simulink library "Lib_EMTAT"  (R2021b)
settings: Solver=VariableStepAuto  StartTime=0.0  StopTime=10.0  RelTol=1e-3
undefined symbols (not defined in the file or in its folder): A_M, B_M, Cj, component_degradation_input, Cs, E0_M, f_sw, K_M, MWS, Q_M, Q_rr, r_c, r_D, R_M, Rj, Ru, SNR_DX_M, SNR_IC_M, SNR_Mn_M, SNR_Mx_M, SOC_Init_M, u_ce0, u_D0
libraries: $bdroot x82, simulink x23, Lib_Dyn_StateSpace_EMTAT x3, PB_Library_Master_Working x1
(part 3 of 7)

== system Lib_EMTAT/Components/Power Flow ==
  note: Add efficiency tables to converters, inverter, and rectifier.
  note: [gcb '/Deg']
  AC-AC Transformer : Subsystem  mask(AC/AC Transformer){X_C_VoltageAC1Vec_M=MWS.I1.Vdc, Y_C_CurrentAC2Vec_M=MWS.I1.Irms, T_C_PowLossArray_M=MWS.I1.Ploss', K=0.0503, FM=0, Plosslim=0}
      mask prompts: X_C_VoltageAC1Vec_M "X_C_VoltageAC1Vec_M - Primary AC Line to Neutral RMS Voltage Vector (X-axis)(nx1)"; Y_C_CurrentAC2Vec_M "Y_C_CurrentAC2Vec_M - Secondary RMS Line Current Vector (Y-axis)(mx1)"; T_C_PowLossArray_M "T_C_PowLossArray_M - Power Loss Table Values (Ploss = f(Irmsout, Vin)(nxm)"; K "Transformer Ratio"; FM "Mode:"; Plosslim "Plosslim - Power Loss Limit, W"
      mask help: This block models an AC/AC transofrmer. The power through the transformer is modified by a user-input power loss table. The primary side is designated as 1. The secondary side is designated as 2.
      settings: AttributesFormatString=AC/AC Transformer
      mask Help:
      | Inputs:
      | 	V_LN_rms_1: Primary line to neutral root-mean-squared alternating current voltage, V_LN_rms (1x1)
      | 	I_L_rms_2: Secondary line root-mean-squared alternating current, A_L_rms (1x1)
      | 	Fail?: Failure toggle (0 = Not failed, 1 = Failed)
      | 	Deg: Decimal percantage of maximum power degredation (0 = New component, 1 = End of life component)
      | Mask Variables:
      | 	X_C_VoltageAC1Vec_M: Primary alternating current line to neutral root-mean-squared voltage vector for power loss map, V_LN_rms (nx1)
      | 	Y_C_CurrentAC2Vec_M: Secondary line root-mean-squared alternating current vector for power loss map, A_LN_rms (nx1)
      | 	T_C_PlossArray_M: Power loss map, W (nxm)
      | 	Failure Modes
      | 		1 - Open circuit.
      | 		2 - Degredation.
      | 	Plosslim: Maximum additional power loss, W (1x1)
      | Outputs:
      | 	V_LN_rms_2: Secondary line to neutral root-mean-squared alternating current voltage, V_LN_rms (1x1)
      | 	Outputs: Low level signals (Bus)
      | 		P_AC_2: Secondary side power, W (1x1)
      | 		P_AC_1: Primary Side power, W (1x1)
      | 		Eff: Efficiency, decimal percentage (1x1)
      | 		V_LN_rms_2: Secondary line to neutral root-mean-squared alternating current voltage, V_LN_rms (1x1)
      | 		V_LN_rms_1: Primary line to neutral root-mean-squared alternating current voltage, V_LN_rms (1x1)
      | 		I_L_rms_2: Secondary line root-mean-squared alternating current, A_L_rms (1x1)
      | 		I_L_rms_1: Primary line root-mean-squared alternating current, I_L_rms (1x1)
      | 		Ploss: Power loss, W (1x1)
      | 	Ploss: Power loss, W (1x1)
      | 	I_L_rms_1: Primary line root-mean-squared alternating current, I_L_rms (1x1)
      mask DialogControl Control3 Prompt: Plot Power Loss Map
      mask DialogControl Control3 Callback:
      | % Plot efficiency map.
      | vals = get_param(gcb,'MaskValues');
      | X = str2num(cell2mat(vals(1)));
      | Y = str2num(cell2mat(vals(2)));
      | Z = str2num(cell2mat(vals(3)));
      | [X,Y] = meshgrid(X,Y);
      | figure('name',[get_param(gcb,'name') ' Power Loss Map'],'numbertitle','off')
      | contour(X,Y,Z,15);
      | xlabel('Voltage In, VDC')
      | ylabel('Line Current Out, A_{rms}')
      | title([get_param(gcb,'name') ' Power Loss Map'])
      | c = colorbar;
      | c.Label.String = 'Power Loss, W';
      mask DialogControl Container3 Prompt: Failure Modes
      mask DialogControl Control2 Prompt: 1 - Open Circuit, 2 - Degradation
  AC-DC Rectifier : Subsystem  mask(Inverter/Rectifier (Source)){X_C_VoltageInVec_M=[0 1000], Y_C_RMSCurrentOutVec_M=[0 1000], T_C_PowLossArray_M=0*ones(2), FM=0, Plosslim=0}
      mask prompts: X_C_VoltageInVec_M "X_C_VoltageInVec_M - DC Voltage Vector (X-axis)(nx1)"; Y_C_RMSCurrentOutVec_M "Y_C_RMSCurrentOutVec_M - RMS Line Current Vector (Y-axis)(mx1)"; T_C_PowLossArray_M "T_C_PowLossArray_M - Power Loss Table Values (Ploss = f(Irmsout, Vin)(nxm)"; FM "Mode:"; Plosslim "Plosslim - Power Loss Limit, W"
      mask help: This block models an inverter/rectifier for use as a power source. The power through the inverter/rectifier is modified by a user-input power loss table.
      settings: AttributesFormatString=AC-DC Rectifier
      mask Help:
      | Inputs:
      | 	V_LN_rms: Line to neutral alternating current voltage, Vrms (1x1)
      | 	I_DC: Direct current, ADC (1x1)
      | 	Fail?: Failure toggle (0 = Not failed, 1 = Failed)
      | 	Deg: Decimal percantage of maximum power degredation (0 = New component, 1 = End of life component)
      | 	I_L_rms(t-1): Line alternating current from one time step delay block, Arms (1x1)
      | Mask Variables:
      | 	X_C_VoltageInVec_M: Direct current voltage vector for efficiency map, VDC (nx1)
      | 	Y_C_RMSCurrentOutVec_M: Line alternating current vector for efficiency map, Irms (mx1)
      | 	T_C_PowLossArray_M: Efficiency matrix, decimal % (nxm)
      | 	K_e: Peak line to line back electromotive force voltage, Vpeak (1x1)
      | 	Failure Modes
      | 		1 - Open circuit.
      | 		2 - Degredation.
      | 	Plosslim: Maximum additional power loss, W (1x1)
      | Outputs:
      | 	V_DC: Direct current voltage, VDC (1x1)
      | 	Outputs: Low level signals (Bus)
      | 		P_AC: Instantaneous alternating current power, W (1x1)
      | 		P_DC: Direct current power, W (1x1)
      | 		Eff: Efficiency, decimal % (1x1)
      | 		V_LN_rms: Line to neutral alternating current voltage, Vrms (1x1)
      | 		V_DC: Direct current voltage, VDC (1x1)
      | 		Vdot_DC: Derivative of direct current voltage, VDC/s (1x1)
      | 		I_L_rms: Line alternating current, Irms (1x1)
      | 		I_DC: Direct current, ADC (1x1)
      | 		Idot_DC: Derivative of direct current, ADC/s (1x1)
      | 		Ploss: Power loss, W (1x1)
      | 	Ploss: Power loss, W (1x1)
      | 	I_L_rms: Line alternating current, Arms (1x1)
      | 	I_L_rms(1): Line alternating current to one time step delay block, Arms (1x1)
      mask DialogControl Control2 Prompt: Plot Power Loss Map
      mask DialogControl Control2 Callback:
      | % Plot efficiency map.
      | vals = get_param(gcb,'MaskValues');
      | X = str2num(cell2mat(vals(1)));
      | Y = str2num(cell2mat(vals(2)));
      | Z = str2num(cell2mat(vals(3)));
      | [X,Y] = meshgrid(X,Y);
      | figure('name',[get_param(gcb,'name') ' Power Loss Map'],'numbertitle','off')
      | contour(X,Y,Z,15);
      | xlabel('Voltage In, VDC')
      | ylabel('Line Current Out, A_{rms}')
      | title([get_param(gcb,'name') ' Power Loss Map'])
      | c = colorbar;
      | c.Label.String = 'Power Loss, W';
      mask DialogControl Container3 Prompt: Failure Modes
      mask DialogControl Control3 Prompt: 1 - Open Circuit, 2 - Degradation
  Cable : Subsystem  mask(Cable){R=0.2}
      mask prompts: R "R_c - Resistance, Ohm"
      mask help: This block models a cable with resistive effects.
      settings: AttributesFormatString=Cable
      mask Help:
      | Inputs:
      | 	Vin: Input voltage, VDC (1x1)
      | 	Iout: Output current, ADC (1x1)
      | 	Fail?: Failure toggle (0 = Not failed, 1 = Failed)
      | 	Iout(t-1): Output curernt from one time step delay block, ADC (1x1)
      | Mask Variables:
      | 	R: Resistance, Ohm (1x1)
      | 	Failure Modes:
      | 		Open circuit failure.
      | Outputs:
      | 	Vout: Output voltage, VDC (1x1)
      | 	Outputs: Low level signals (Bus)
      | 		Pout: Electrical power out, W (1x1)
      | 		Pin: Electrical power in, W (1x1)
      | 		Iin: Input current, ADC (1x1)
      | 		Iout: Output current, ADC (1x1)
      | 		Vin: Input voltage, VDC (1x1)
      | 		Vout: Output voltage, VDC (1x1)
      | 		R: Resistance, Ohm (1x1)
      | 		Ploss: Power loss due to resistive effects, W (1x1)
      | 	Ploss: Power loss due to resistive effects, W (1x1)
      | 	Iin: Input current, ADC (1x1)
      | 	Iout(t): Output current to one time step delay block, ADC (1x1)
      mask DialogControl Container3 Prompt: Failure Modes
      mask DialogControl Control2 Prompt: Mode: Open Circuit
  Current Distribution : Subsystem  mask(Current Distribution){}
      settings: AttributesFormatString=Current Distribution
  Current Junction : Subsystem  mask(Current Junction){Nb=3}
      mask prompts: Nb "Nb - # of branches"
      mask help: This block adds a vector of input currents (I).
      settings: AttributesFormatString=Current Junction
      mask Help:
      | Inputs:
      | 	I: Currents to be summed, ADC (nx1)
      | Outputs:
      | 	Isum: Net current, ADC (1x1)
      mask DialogControl Control2 Prompt: Note: There is no limit to the number of multiplexed currents.
      mask DialogControl Container2 Prompt: Parameters
  DC-AC Inverter : Subsystem  mask(Inverter/Rectifier (Sink)){X_C_VoltageInVec_M=[0 1000], Y_C_RMSCurrentOutVec_M=[0 1000], T_C_PowLossArray_M=zeros(2), K_e=0.0503, FM=0, Plosslim=0}
      mask prompts: X_C_VoltageInVec_M "X_C_VoltageInVec_M - DC Voltage Vector (X-axis)(nx1)"; Y_C_RMSCurrentOutVec_M "Y_C_RMSCurrentOutVec_M - RMS Line Current Vector (Y-axis)(mx1)"; T_C_PowLossArray_M "T_C_PowLossArray_M - Power Loss Table Values (Ploss = f(Irmsout, Vin)(nxm)"; K_e "K_e - Back EMF Constant, V_LL_peak/RPM"; FM "Mode:"; Plosslim "Plosslim - Power Loss Limit, W"
      mask help: This block models an inverter/rectifier for use as a power sink. The power through the inverter/rectifier is modified by a user-input efficiency table.
      settings: AttributesFormatString=DC-AC Inverter
      mask Help:
      | Inputs:
      | 	V_DC: Direct current voltage, VDC (1x1)
      | 	N: Shaft speed, RPM (1x1)
      | 	I_L_rms: Line alternating current, Arms (1x1)
      | 	Fail?: Failure toggle (0 = Not failed, 1 = Failed)
      | 	Deg: Decimal percantage of maximum power degredation (0 = New component, 1 = End of life component)
      | Mask Variables:
      | 	X_C_VoltageInVec_M: Direct current voltage vector for efficiency map, VDC (nx1)
      | 	Y_C_RMSCurrentOutVec_M: Line alternating current vector for efficiency map, Irms (mx1)
      | 	T_C_PowLossArray_M: Efficiency matrix, decimal % (nxm)
      | 	K_e: Peak line to line back electromotive force voltage, Vpeak (1x1)
      | 	Failure Modes
      | 		1 - Open circuit.
      | 		2 - Degredation.
      | 	Plosslim: Maximum additional power loss, W (1x1)
      | Outputs:
      | 	V_LN_rms: Line to neutral alternating current voltage, Vrms (1x1)
      | 	Outputs: Low level signals (Bus)
      | 		P_AC: Instantaneous alternating current power, W (1x1)
      | 		P_DC: Direct current power, W (1x1)
      | 		Eff: Efficiency, decimal % (1x1)
      | 		V_LN_rms: Line to neutral alternating current voltage, Vrms (1x1)
      | 		V_DC: Direct current voltage, VDC (1x1)
      | 		Vdot_DC: Derivative of direct current voltage, VDC/s (1x1)
      | 		I_L_rms: Line alternating current, Irms (1x1)
      | 		I_DC: Direct current, ADC (1x1)
      | 		Idot_DC: Derivative of direct current, ADC/s (1x1)
      | 		Ploss: Power loss, W (1x1)
      | 	Ploss: Power loss, W (1x1)
      | 	I_DC: Direct current, ADC (1x1)
      mask DialogControl Control3 Prompt: Plot Power Loss Map
      mask DialogControl Control3 Callback:
      | % Plot efficiency map.
      | vals = get_param(gcb,'MaskValues');
      | X = str2num(cell2mat(vals(1)));
      | Y = str2num(cell2mat(vals(2)));
      | Z = str2num(cell2mat(vals(3)));
      | [X,Y] = meshgrid(X,Y);
      | figure('name',[get_param(gcb,'name') ' Power Loss Map'],'numbertitle','off')
      | contour(X,Y,Z,15);
      | xlabel('Voltage In, VDC')
      | ylabel('Line Current Out, A_{rms}')
      | title([get_param(gcb,'name') ' Power Loss Map'])
      | c = colorbar;
      | c.Label.String = 'Power Loss, W';
      mask DialogControl Container3 Prompt: Failure Modes
      mask DialogControl Control2 Prompt: 1 - Open Circuit, 2 - Degradation
  DC-DC Converter (Set Output Voltage) : Subsystem  mask(DC-DC Converter (Set Output Voltage)){X_Vin_VoltageVec_M=[0 100 1000 5000], Y_Iout_CurrentVec_M=[0 10 100 150], T_C_PlossArray_M=0.98*ones(4,4), FM=0, Plosslim=0}
      mask prompts: X_Vin_VoltageVec_M "X_Vin_VoltageVec_M - Efficiency Table Voltage In Vector (X-axis)(nx1)"; Y_Iout_CurrentVec_M "Y_Iout_CurrentVec_M - Efficiency Table Current Out Vector (Y-axis)(mx1)"; T_C_PlossArray_M "T_C_PlossArray_M - Power Loss Table Values (Eff = f(i, V)(nxm)"; FM "Mode:"; Plosslim "Plosslim - Power Loss Limit, W"
      mask help: This block models the power flow through a DC-DC converter using a user specified power loss table. The output voltage (Vout) can also be set using variable Vset.
      settings: AttributesFormatString=|
      | DC-DC Converter
      | (Set Output Voltage)
      mask Help:
      | Inputs:
      | 	Vset: Voltage setpoint, VDC (1x1)
      | 	Vin: Input voltage, VDC (1x1)
      | 	Iout: Output current, ADC (1x1)
      | 	Fail?: Failure toggle (0 = Not failed, 1 = Failed)
      | 	Deg: Decimal percantage of maximum power degredation (0 = New component, 1 = End of life component)
      | Mask Variables:
      | 	X_Vin_VoltageVec_M: Input voltage vector for power loss map, VDC (nx1)
      | 	Y_Iout_CurrentVec_M: Output current vector for power loss map, ADC (mx1)
      | 	T_C_PlossArray_M: Power loss map, W (nxm)
      | 	Failure Modes
      | 		1 - Open circuit.
      | 		2 - Degredation.
      | 	Plosslim: Maximum additional power loss, W (1x1)
      | Outputs:
      | 	Vout: Output voltage, VDC (1x1)
      | 	Outputs: Low level signals (Bus)
      | 		Pin: Input power, W (1x1)
      | 		Pout: Output power, W (1x1)
      | 		Eff: Efficiency, decimal % (1x1)
      | 		Vout: Output voltage, VDC (1x1)
      | 		Vdotout: Derivative of output voltage, VDC/s (1x1)
      | 		Vin: Input voltage, VDC (1x1)
      | 		Vdotin: Derivative of input voltage, VDC/s (1x1)
      | 		Iin: Input current, ADC (1x1)
      | 		Idotin: Derivative of input current, ADC/s (1x1)
      | 		Iout: Output current, ADC (1x1)
      | 		Idotout: Derivative of output current, ADC/s (1x1)
      | 		Ploss: Power loss, W (1x1)
      | 		Vset: Voltage setpoint, VDC (1x1)
      | 	Ploss: Power loss, W (1x1)
      | 	Iin: Input current, ADC (1x1)
      mask DialogControl Control3 Prompt: Plot Power Loss Map
      mask DialogControl Control3 Callback:
      | % Plot power loss map.
      | vals = get_param(gcb,'MaskValues');
      | X = str2num(cell2mat(vals(1)));
      | Y = str2num(cell2mat(vals(2)));
      | Z = str2num(cell2mat(vals(3)));
      | [X,Y] = meshgrid(X,Y);
      | figure('name',[get_param(gcb,'name') ' Power Loss Map'],'numbertitle','off')
      | contour(X,Y,Z,15);
      | xlabel('Voltage In, VDC')
      | ylabel('Current Out, ADC')
      | title([get_param(gcb,'name') ' Power Loss Map'])
      | c = colorbar;
      | c.Label.String = 'Power loss, W';
      mask DialogControl Container3 Prompt: Failure Modes
      mask DialogControl Control2 Prompt: 1 - Open Circuit, 2 - Degradation
  DC-DC Converter (Regulate Output Voltage) : Subsystem  mask(DC-DC Converter (Regulate Output Voltage)){X_Vin_VoltageVec_M=[0 100 1000 5000], Y_Iout_CurrentVec_M=[0 10 100 150], T_C_PlossArray_M=0.98*ones(4,4), FM=0, Plosslim=0}
      mask prompts: X_Vin_VoltageVec_M "X_Vin_VoltageVec_M - Efficiency Table Voltage In Vector (X-axis)(nx1)"; Y_Iout_CurrentVec_M "Y_Iout_CurrentVec_M - Efficiency Table Current Out Vector (Y-axis)(mx1)"; T_C_PlossArray_M "T_C_PlossArray_M - Power Loss Table Values (Eff = f(i, V)(nxm)"; FM "Mode:"; Plosslim "Plosslim - Power Loss Limit, W"
      mask help: This block models the power flow through a DC-DC converter using a user specified efficiency table. The output voltage (Vout) can also be set using variable Vset.
      settings: AttributesFormatString=|
      | DC-DC Converter
      | (Regulate Output Voltage)
      mask Help:
      | Inputs:
      | 	Vout: Output voltage, VDC (1x1)
      | 	Vin: Input voltage, VDC (1x1)
      | 	Ioutdmd: Output current demand, ADC (1x1)
      | 	Fail?: Failure toggle (0 = Not failed, 1 = Failed)
      | 	Deg: Decimal percantage of maximum power degredation (0 = New component, 1 = End of life component)
      | Mask Variables:
      | 	X_Vin_VoltageVec_M: Input voltage vector for power loss map, VDC (nx1)
      | 	Y_Iout_CurrentVec_M: Output current vector for power loss map, ADC (mx1)
      | 	T_C_PlossArray_M: Power loss map, W (nxm)
      | 	Failure Modes
      | 		1 - Open circuit.
      | 		2 - Degredation.
      | 	Plosslim: Maximum additional power loss, W (1x1)
      | Outputs:
      | 	Outputs: Low level signals (Bus)
      | 		Pin: Input power, W (1x1)
      | 		Pout: Output power, W (1x1)
      | 		Eff: Efficiency, decimal % (1x1)
      | 		Vout: Output voltage, VDC (1x1)
      | 		Vdotout: Derivative of output voltage, VDC/s (1x1)
      | 		Vin: Input voltage, VDC (1x1)
      | 		Vdotin: Derivative of input voltage, VDC/s (1x1)
      | 		Iin: Input current, ADC (1x1)
      | 		Idotin: Derivative of input current, ADC/s (1x1)
      | 		Iout: Output current, ADC (1x1)
      | 		Idotout: Derivative of output current, ADC/s (1x1)
      | 		Ploss: Power loss, W (1x1)
      | 	Ploss: Power loss, W (1x1)
      | 	Iin: Input current, ADC (1x1)
      | 	Iout: Output current, ADC (1x1)
      mask DialogControl Control3 Prompt: Plot Power Loss Map
      mask DialogControl Control3 Callback:
      | % Plot power loss map.
      | vals = get_param(gcb,'MaskValues');
      | X = str2num(cell2mat(vals(1)));
      | Y = str2num(cell2mat(vals(2)));
      | Z = str2num(cell2mat(vals(3)));
      | [X,Y] = meshgrid(X,Y);
      | figure('name',[get_param(gcb,'name') ' Power Loss Map'],'numbertitle','off')
      | contour(X,Y,Z,15);
      | xlabel('Voltage In, VDC')
      | ylabel('Current Out, ADC')
      | title([get_param(gcb,'name') ' Power Loss Map'])
      | c = colorbar;
      | c.Label.String = 'Power loss, W';
      mask DialogControl Container3 Prompt: Failure Modes
      mask DialogControl Control2 Prompt: 1 - Open Circuit, 2 - Degradation
  Electrical Bus : Subsystem  mask(Bus){C=6e-3, Nb=0}
      mask prompts: C "C - Capacitance, F"; Nb "Nb - # of branches"
      mask help: This block represents an electrical bus with capacitance effects.
      settings: AttributesFormatString=Electrical Bus
      mask Help:
      | Inputs:
      | 	I: Curents to be summed, ADC (nx1)
      | 	V: Voltage from integrator block, VDC (1x1)
      | Mask Variables:
      | 	C: Capacitance, F (1x1)
      | Outputs:
      | 	V: Bus voltage, VDC (1x1)
      | 	Vdot: Derivative of bus voltage to integrator block, VDC/s (1x1)
  Energy Storage Device : Subsystem  mask(Energy Storage Device){C=130, ESR=0.02, TSE=69, BlkNm=double(gcb)}
      mask prompts: C "C - Capacitance, F"; ESR "ESR - Equivilent Series Resistance, Ohm"; TSE "TSE - Max Stored Energy, W-h"; BlkNm "Block Name"
      mask help: This block models a capacitor with equivilent series resistive (ESR) effects.
      mask init:
      | BN = gcb;
      settings: AttributesFormatString=Energy Storage Device
      mask Help:
      | Inputs:
      | 	Iout: Output current, ADC (1x1)
      | 	V: Voltage from integrator block, V (1x1)
      | 	Iout(t-1): Output current from one time step delay block, ADC (1x1)
      | Mask Variables:
      | 	C - Capacitance, F (1x1)
      | 	ESR - Equivilent Series Resistance, Ohm (1x1)
      | 	TSE - Max Stored Energy, W-h (1x1)
      | Outputs:
      | 	Vout: Output Voltage, VDC (1x1)
      | 	Outputs: Lower level signals (Bus)
      | 		E: Energy, W-h (1x1)
      | 		Iout: Output current, ADC (1x1)
      | 		Idotout: Derivative of output current, ADC/s (1x1)
      | 		Vout: Output Voltage, VDC (1x1)
      | 		Vdotout: Derivative of output voltage, VDC/s (1x1)
      | 		SOC: State of charge, % (1x1)
      | 		SOCdot: Derivative of state of charge, %/s (1x1)
      | 		Ploss: Power loss due to resistive effects, W (1x1)
      | 	Ploss: Power loss due to resistive effects, W (1x1)
      | 	Vdot: Derivative of output voltage to integrator block, VDC/s (1x1)
      | 	Iout(t): Output current to one time step delay block, ADC (1x1)
  Mechanical Shaft : Subsystem  mask(Mechanical Shaft){J=0.01, B=0.001}
      mask prompts: J "J - Inertia, lb-ft-s^2"; B "B - Damping, lb-ft-s"
      mask help: This block models a mechanical shaft with inertial and viscous damping effects.
      settings: AttributesFormatString=Mechanical Shaft
      mask Help:
      | Inputs:
      | 	T: Torques to be summed, lbf-ft (nx1)
      | 	Fail?: Failure toggle (0 = Not failed, 1 = Failed)
      | 	N: Shaft speed, RPM (1x1)
      | Mask Variables:
      | 	J: Inertia, lbf-ft-s^2 or slug-ft^2 (1x1)
      | 	B: Viscous damping coefficient, lbf-ft-s (1x1)
      | 	Failure Modes:
      | 		Shaft break.
      | Outputs:
      | 	Outputs: Low level signals (Bus):
      | 		Tnet: Net shaft torque, lbf-ft (1x1)
      | 		N: Shaft speed, RPM (1x1)
      | 		Ndot: Acceleration to integrator block, RPM/s (1x1)
      | 		Heat: Heat from viscous friction, Btu (1x1)
      | 		SBFail: Shaft break failure (0 = Not failed, 1 = Failed)
      | 	Heat: Heat from viscous friction, Btu (1x1)
      | 	Ndot: Acceleration to integrator block, RPM/s (1x1)
      mask DialogControl Container3 Prompt: Failure Mode
      mask DialogControl Control2 Prompt: Mode: Shaft Break
  Power Supply (Set Voltage) : Subsystem  mask(Power Supply (Set Voltage)){Nb=0}
      mask prompts: Nb "Nb - # of branches"
      mask help: This block models a power supply that uses Vset to set, not regulate, the bus voltage based on a vector of current demands (Idmd).
      settings: AttributesFormatString=|
      | Power Supply
      | (Set Voltage)
      mask Help:
      | Inputs:
      | 	Vset: Voltage setpoint, VDC (1x1)
      | 	Idmd: Current demand, ADC (nx1)
      | Outputs:
      | 	Outputs: Low level signals (Bus)
      | 		Vout: Output Voltage, VDC (1x1)
      | 		Idmdsum: Sum of vector of current demands, ADC (1x1)
      | 		Pdmd: Power demand, W (1x1)
      | 	Vout: Output Voltage, VDC (1x1)
      mask DialogControl Container2 Prompt: Parameters
  Resistive Load Bank : Subsystem  ClipboardFcn=|  mask(Active Resistor){}
      | Active Resistor
      | Version: %<LibraryVersion>
      mask help: This block changes its resistance (R) based on a power command (Pset) to produce a current demand (Iin).
      settings: AttributesFormatString=Resistive Load Bank
      mask Help:
      | Inputs:
      | 	V: Voltage, VDC (1x1)
      | 	Pset: Power setpoint, W (1x1)
      | 	Fail?: Failure toggle (0 = Not failed, 1 = Failed)
      | Mask Variables:
      | 	Faulure Modes:
      | 		Open circuit failure.
      | Outputs:
      | 	Outputs: Low level signals (Bus)
      | 		V: Voltage, VDC (1x1)
      | 		I: Current, ADC (1x1)
      | 		Pset: Power setpoint, W (1x1)
      | 		R: Resistance, Ohm (1x1)
      | 		Ploss: Power loss due to resistive effects, W (1x1)
      | 	Ploss: Power loss due to resistive effects, W (1x1)
      | 	Iin: Input current, ADC (1x1)
      mask DialogControl Container2 Prompt: Failure Modes
      mask DialogControl Control2 Prompt: Mode: Open Circuit
  Three Phase Electric Machine (Sink) : Subsystem  mask(Three Phase Electric Machine (Sink)){X_C_SpeedVec_M=[0 8000], Y_C_TorqueVec_M=[0 300], T_C_EffArray_M=[0.97 0.95; 0.93 0.94], FM=0}
      mask prompts: X_C_SpeedVec_M "X_C_SpeedVec_M - Efficiency Table Speed Vector (X-axis)(nx1)"; Y_C_TorqueVec_M "Y_C_TorqueVec_M - Efficiency Table Torque Vector (Y-axis)(mx1)"; T_C_EffArray_M "T_C_EffArray_M - Efficiency Table Values (Eff = f(i, V)(nxm)"; FM "Mode:"
      mask help: This block models an three phase motor/generator for use as a power sink. The power through the motor/generator is modified by a user-input efficiency table.
      settings: AttributesFormatString=|
      | Three Phase Electric Machine
      | (Sink)
      mask Help:
      | Inputs:
      | 	V_LN_rms: Line to neutral alternating current voltage, Vrms (1x1)
      | 	N: Shaft speed, RPM (1x1)
      | 	T*: Torque setpoint, lbf-ft (1x1)
      | 	Fail?: Failure toggle (0 = Not failed, 1 = Failed)
      | 	Deg: Decimal percantage of maximum power degredation (0 = New component, 1 = End of life component)
      | Mask Variables:
      | 	X_C_VoltageInVec_M: Direct current voltage vector for efficiency map, VDC (nx1)
      | 	Y_C_RMSCurrentOutVec_M: Line alternating current vector for efficiency map, Irms (mx1)
      | 	T_C_PowLossArray_M: Efficiency matrix, decimal % (nxm)
      | 	K_e: Peak line to line back electromotive force voltage, Vpeak (1x1)
      | 	Failure Modes
      | 		1 - Open circuit.
      | 		2 - Degredation.
      | 	Plosslim: Maximum additional power loss, W (1x1)
      | Outputs:
      | 	T: Torque, lbf-ft (1x1)
      | 	Outputs: Low level signals (Bus)
      | 		P_mech: Mechanical power, W (1x1)
      | 		P_elec: Electrical power, W (1x1)
      | 		Eff: Efficiency, decimal % (1x1)
      | 		I_L_rms: Line alternating current, Irms (1x1)
      | 		V_LN_rms: Line to neutral alternating current voltage, Vrms (1x1)
      | 		N: Shaft speed, RPM (1x1)
      | 		T: Torque, lbf-ft (1x1)
      | 		Ploss: Power loss, W (1x1)
      | 		T*: Torque setpoint, lbf-ft (1x1)
      | 		Tdot: Derivative of torque, lbf-ft/s (1x1)
      | 		OCFail: Open circuit failure (0 = No fail, 1 = Fail)
      | 		DegFail: Degredation failure (0 = No fail, 1 = Fail)
      | 	Ploss: Power loss, W (1x1)
      | 	I_L_rms: Line alternating current, Arms (1x1)
      mask DialogControl Container2 Prompt: Parameters
      mask DialogControl Plot Prompt: Plot Efficiency Map
      mask DialogControl Plot Callback:
      | % Plot efficiency map.
      | vals = get_param(gcb,'MaskValues');
      | X = str2num(cell2mat(vals(1)));
      | Y = str2num(cell2mat(vals(2)));
      | Z = str2num(cell2mat(vals(3)));
      | [X,Y] = meshgrid(X,Y);
      | figure('name',[get_param(gcb,'name') ' Efficiency Map'],'numbertitle','off')
      | contour(X,Y,Z,15);
      | xlabel('Speed, RPM')
      | ylabel('Torque, lbf-ft')
      | title([get_param(gcb,'name') ' Efficiency Map'])
      | c = colorbar;
      | c.Label.String = 'Efficiency';
      mask DialogControl Container3 Prompt: Failure Modes
      mask DialogControl Control3 Prompt: 1 - Open Circuit, 2 - Degradation
  Three Phase Electric Machine (Source) : Subsystem  mask(Three Phase Electric Machine (Source)){X_C_SpeedVec_M=[0 10000], Y_C_TorqueVec_M=[0 500], T_C_EffArray_M=0.9*ones(2), Ke=0.05, FM=0}
      mask prompts: X_C_SpeedVec_M "X_C_SpeedVec_M - Efficiency Table Speed Vector (X-axis)(nx1)"; Y_C_TorqueVec_M "Y_C_TorqueVec_M - Efficiency Table Torque Vector (Y-axis)(mx1)"; T_C_EffArray_M "T_C_EffArray_M - Efficiency Table Values (Eff = f(i, V)(nxm)"; Ke "Ke - Back EMF Constant, V_LL_peak/RPM"; FM "Mode:"
      mask help: This block models an motor/generator for use as a power source. The power through the motor/generator is modified by a user-input efficiency table.
      settings: AttributesFormatString=|
      | Three Phase Electric Machine
      | (Source)
      mask Help:
      | Inputs:
      | 	N: Shaft speed, RPM (1x1)
      | 	I_L_rms: Line alternating current, Arms (1x1)
      | 	Fail?: Failure toggle (0 = Not failed, 1 = Failed)
      | 	Deg: Decimal percentage of maximum power degredation (0 = New component, 1 = End of life component)
      | 	T(t-1): Torque from one time step delay block, lbf-ft (1x1)
      | Mask Variables:
      | 	X_C_VoltageInVec_M: Direct current voltage vector for efficiency map, VDC (nx1)
      | 	Y_C_RMSCurrentOutVec_M: Line alternating current vector for efficiency map, Irms (mx1)
      | 	T_C_PowLossArray_M: Efficiency matrix, decimal % (nxm)
      | 	K_e: Peak line to line back electromotive force voltage, Vpeak (1x1)
      | 	Failure Modes
      | 		1 - Open circuit.
      | 		2 - Degredation.
      | 	Plosslim: Maximum additional power loss, W (1x1)
      | Outputs:
      | 	V_LN_rms: Line to neutral alternating current voltage, Vrms (1x1)
      | 	T: Torque, lbf-ft (1x1)
      | 	Outputs: Low level signals (Bus)
      | 		P_mech: Mechanical power, W (1x1)
      | 		P_elec: Electrical power, W (1x1)
      | 		Eff: Efficiency, decimal % (1x1)
      | 		N: Shaft speed, RPM (1x1)
      | 		T: Torque, lbf-ft (1x1)
      | 		Tdot: Derivative of torque, lbf-ft/s (1x1)
      | 		I_L_rms: Line alternating current, Irms (1x1)
      | 		V_LN_rms: Line to neutral alternating current voltage, Vrms (1x1)
      | 		Ploss: Power loss, W (1x1)
      | 		OCFail: Open circuit failure (0 = No fail, 1 = Fail)
      | 		DegFail: Degredation failure (0 = No fail, 1 = Fail)
      | 	Ploss: Power loss, W (1x1)
      | 	T(t): Torque to one time step delay block, lbf-ft (1x1)
      mask DialogControl Control2 Prompt: Plot Efficiency Map
      mask DialogControl Control2 Callback:
      | % Plot efficiency map.
      | vals = get_param(gcb,'MaskValues');
      | X = str2num(cell2mat(vals(1)));
      | Y = str2num(cell2mat(vals(2)));
      | Z = str2num(cell2mat(vals(3)));
      | [X,Y] = meshgrid(X,Y);
      | figure('name',[get_param(gcb,'name') ' Efficiency Map'],'numbertitle','off')
      | contour(X,Y,Z,15);
      | xlabel('Speed, RPM')
      | ylabel('Torque, lbf-ft')
      | title([get_param(gcb,'name') ' Efficiency Map'])
      | c = colorbar;
      | c.Label.String = 'Efficiency';
      mask DialogControl Container3 Prompt: Failure Modes
      mask DialogControl Control3 Prompt: 1 - Open Circuit, 2 - Degradation

== system Lib_EMTAT/Extras/Exergy (Heat) ==
  note: X = Q - m*Cp*dTamb
  Heat : Inport
  dTamb : Inport  Port=2
  Divide : Product  Inputs=***
  Joules to BTU : Gain  Gain=0.000947817
  Mass (lbm) : Constant  Value=m
  Specific Heat (Btu/lbm-degF) : Constant  Value=Cp
  Sum : Sum  Inputs=|+-
  Exergy : Outport
  wires:
  Joules to BTU/1 -> Sum/1
  Heat/1 -> Joules to BTU/1
  dTamb/1 -> Divide/1
  Mass (lbm)/1 -> Divide/2
  Specific Heat (Btu/lbm-degF)/1 -> Divide/3
  Divide/1 -> Sum/2
  Sum/1 -> Exergy/1

== system Lib_EMTAT/Extras/Exergy (Ploss) ==
  note: X = Q - m*Cp*dTamb
  Ploss : Inport
  dTamb : Inport  Port=2
  Divide : Product  Inputs=***
  Integrator : Integrator  InitialCondition=Qo/0.000947817
  Joules to BTU : Gain  Gain=0.000947817
  Mass (lbm) : Constant  Value=m
  Specific Heat (Btu/lbm-degF) : Constant  Value=Cp
  Sum : Sum  Inputs=|+-
  Exergy : Outport
  wires:
  Sum/1 -> Exergy/1
  Divide/1 -> Sum/2
  Specific Heat (Btu/lbm-degF)/1 -> Divide/3
  Mass (lbm)/1 -> Divide/2
  dTamb/1 -> Divide/1
  Ploss/1 -> Integrator/1
  Integrator/1 -> Joules to BTU/1
  Joules to BTU/1 -> Sum/1

== system Lib_EMTAT/Extras/Temperature (Heat) ==
  Heat : Inport
  dTamb : Inport  Port=2
  Tamb : Inport  Port=3
  Divide : Product  Inputs=*//
  Joules to BTU : Gain  Gain=0.000947817
  Mass (lbm) : Constant  Value=m
  Specific Heat (Btu/(lbm-degF)) : Constant  Value=Cp
  Sum : Sum  Inputs=|++
  Sum1 : Sum  Inputs=|++
  Temp : Outport
  wires:
  Joules to BTU/1 -> Divide/1
  Heat/1 -> Joules to BTU/1
  Divide/1 -> Sum/1
  Sum1/1 -> Sum/2
  Sum/1 -> Temp/1
  Mass (lbm)/1 -> Divide/2
  Specific Heat (Btu/(lbm-degF))/1 -> Divide/3
  Tamb/1 -> Sum1/2
  dTamb/1 -> Sum1/1

== system Lib_EMTAT/Extras/Temperature (Ploss) ==
  Ploss : Inport
  dTamb : Inport  Port=2
  Tamb : Inport  Port=3
  Divide : Product  Inputs=*//
  Integrator : Integrator  InitialCondition=Qo/0.000947817
  Joules to BTU : Gain  Gain=0.000947817
  Mass (lbm) : Constant  Value=m
  Specific Heat (Btu/(lbm-degF)) : Constant  Value=Cp
  Sum : Sum  Inputs=|++
  Sum1 : Sum  Inputs=|++
  Temp : Outport
  wires:
  dTamb/1 -> Sum1/1
  Tamb/1 -> Sum1/2
  Specific Heat (Btu/(lbm-degF))/1 -> Divide/3
  Mass (lbm)/1 -> Divide/2
  Sum/1 -> Temp/1
  Sum1/1 -> Sum/2
  Divide/1 -> Sum/1
  Integrator/1 -> Joules to BTU/1
  Joules to BTU/1 -> Divide/1
  Ploss/1 -> Integrator/1

== system Lib_EMTAT/Loop Blocks/Outer Loop Integrator ==
  Xdot : Inport
  Constant : Constant  Value=Xo
  Integrator : Integrator  InitialConditionSource=external
  X : Outport
  wires:
  Integrator/1 -> X/1
  Xdot/1 -> Integrator/1
  Constant/1 -> Integrator/2

== system Lib_EMTAT/Loop Blocks/Outer Loop Time Step Delay ==
  W(t) : Inport
  Unit Delay : UnitDelay  InitialCondition=Wo  SampleTime=-1  HasFrameUpgradeWarning=on
  W(t-1) : Outport
  wires:
  W(t)/1 -> Unit Delay/1
  Unit Delay/1 -> W(t-1)/1

== system Lib_EMTAT/Numerical Methods/Jacobian Calculator ==
  Reset : Inport  PortDimensions=1
  f(x_p) : Inport  Port=2  PortDimensions=size(N_Per_M,2)
  Xo : Inport  Port=3  PortDimensions=size(N_Per_M,2)
  Constant2 : Constant  Value=N_Per_M
  Counter : Subsystem  mask{N_Ind_M=prod(size(N_Per_M))}
      mask prompts: N_Ind_M "number of independents, N_Ind_M"
  Jacobian : Subsystem
  Terminator : Terminator
  J : Outport  PortDimensions=[size(N_Per_M,2), size(N_Per_M,2)]
  x_p : Outport  Port=2  PortDimensions=size(N_Per_M,2)
  Iteration : Outport  Port=3  PortDimensions=1
  Active : Outport  Port=4  PortDimensions=1
  inv(J) : Outport  Port=5  PortDimensions=[size(N_Per_M,2), size(N_Per_M,2)]
  JacFailed : Outport  Port=6  PortDimensions=1
  wires:
  f(x_p)/1 -> Jacobian/3(f(x_p))
  Constant2/1 -> Jacobian/2(Per)
  Jacobian/1(x_p) -> x_p/1
  Reset/1 -> Counter/1(Reset)
  Counter/1(Enable) -> Active/1, Jacobian/Enable
  Xo/1 -> Jacobian/4(Xo)
  Counter/2(Iteration) -> Iteration/1, Jacobian/1(Iteration)
  Jacobian/2(Inv(J)) -> inv(J)/1
  Jacobian/3(J) -> J/1
  Jacobian/4(y_State) -> Terminator/1
  Jacobian/5(JacFailed) -> JacFailed/1

== system Lib_EMTAT/Numerical Methods/Newton Raphson Solver ==
  Enable : Inport  PortDimensions=1
  inv(f'(x(n))) : Inport  Port=2  PortDimensions=[length(NR_IC_M),length(NR_IC_M)]
  f(x(n)) : Inport  Port=3  PortDimensions=length(NR_IC_M)
  NR Update : Subsystem
  Switch : Switch  Criteria=u2 > Threshold
  Unit Delay : UnitDelay  InitialCondition=NR_IC_M  SampleTime=-1  HasFrameUpgradeWarning=on
  x(n) : Outport  PortDimensions=length(NR_IC_M)
  x(n+1) : Outport  Port=2  PortDimensions=length(NR_IC_M)
  wires:
  NR Update/1(x(n+1)) -> Switch/1
  inv(f'(x(n)))/1 -> NR Update/2(inv(J))
  f(x(n))/1 -> NR Update/1(f(x))
  Switch/1 -> x(n+1)/1, Unit Delay/1
  Enable/1 -> NR Update/Enable, Switch/2
  Unit Delay/1 -> NR Update/3(x(n)), Switch/3, x(n)/1

== system Lib_EMTAT/Solvers/Iterative NR Solver w JacobianCalc ==
  Iterations : Inport  PortDimensions=1
  Enable : Inport  Port=2  PortDimensions=1
  f(x) : Inport  Port=3  PortDimensions=length(SNR_IC_M)
  Bus Creator : BusCreator  Inputs=2
  JC w Reset : Subsystem
  Logical Operator : Logic  AllPortsSameDT=off  OutDataTypeStr=boolean
  NRwCond : Subsystem
  do_while Condition : Outport  PortDimensions=1
  X : Outport  Port=2  PortDimensions=length(SNR_IC_M)
  S_Data : Outport  Port=3
  wires:
  f(x)/1 -> NRwCond/1(f(x)), JC w Reset/1(f(x))
  NRwCond/1(CCnd) -> Logical Operator/2
  Iterations/1 -> JC w Reset/2(Iter)
  NRwCond/2(x(n+1)) -> JC w Reset/3(x(n+1))
  JC w Reset/1(J) -> Bus Creator/1
  JC w Reset/3(X_out) -> X/1
  JC w Reset/4(JC_Active) -> NRwCond/2(JC_Active)
  JC w Reset/5(inv(J)) -> NRwCond/3(inv(f'(x)))
  Enable/1 -> JC w Reset/Enable, NRwCond/Enable, Logical Operator/1
  Logical Operator/1 -> do_while Condition/1
  Bus Creator/1 -> S_Data/1
  JC w Reset/2(JacFailed) -> Bus Creator/2

== system Lib_EMTAT/Solvers/SS NR Solver w JacobianCalc  ==
  Enable : Inport  PortDimensions=1
  f(x) : Inport  Port=2  PortDimensions=length(SNR_IC_M)
  Bus Creator : BusCreator  Inputs=3
  JacCalc w Reset : Subsystem  TreatAsAtomicUnit=on
  NewRaph w Cond : Subsystem  TreatAsAtomicUnit=on
  X : Outport  PortDimensions=length(SNR_IC_M)
  S_Data : Outport  Port=2  PortDimensions={1,[length(SNR_IC_M),length(SNR_IC_M)]}
  wires:
  JacCalc w Reset/1(X_out) -> X/1
  JacCalc w Reset/2(JC_Active) -> NewRaph w Cond/2(JC_Active)
  JacCalc w Reset/3(inv(J)) -> NewRaph w Cond/3(inv(f'x(n)))
  JacCalc w Reset/4(J) -> [J]
  NewRaph w Cond/2(CCnd) -> JacCalc w Reset/2(CCnd)
  f(x)/1 -> NewRaph w Cond/1(f(x(n))), JacCalc w Reset/1(f(x))
  NewRaph w Cond/3(x(n+1)) -> JacCalc w Reset/3(x(n+1))
  NewRaph w Cond/1(Converged) -> Bus Creator/1  "Converged"
  Enable/1 -> NewRaph w Cond/Enable, JacCalc w Reset/Enable
  JacCalc w Reset/5(JacFailed) -> [JacFailed]
  Bus Creator/1 -> S_Data/1
  [J] -> Bus Creator/2  "J"
  [JacFailed] -> Bus Creator/3  "JacFailed"

== system Lib_EMTAT/Components/Physics-Based/Boost Converter ==
  Vin : Inport
  x : Inport  Port=2
  d : Inport  Port=3
  dt : Inport  Port=4
  Iout : Inport  Port=5
  Temp (Rankine) : Inport  Port=6  Unit=degC
  FaultToggle : Inport  Port=7
  Bus Creator : BusCreator  Inputs=11
  Catastrophic Fault Block{,1..6} (7 alike) : $bdroot/Components/Physics-Based/Catastrophic Fault Block  SystemSampleTime=-1  VariantActivationTime=update diagram  Latency=0  AutoFrameSizeCalculation=off
  DC - DC Converter : Subsystem
  Display : Display
  Divide : Product  Inputs=*/
  Divide1 : Product  Inputs=*/
  "Power Loss " : Subsystem
  Product1 : Product
  Product3 : Product
  Rankine to Celsius : $bdroot/Components/Physics-Based/Rankine to Celsius  SystemSampleTime=-1  VariantActivationTime=update diagram  Latency=0  AutoFrameSizeCalculation=off
  Switch : Switch  Criteria=u2 > Threshold
  Voltage Catastrophic Fault Block : $bdroot/Components/Physics-Based/Voltage Catastrophic Fault Block  SystemSampleTime=-1  VariantActivationTime=update diagram  Latency=0  AutoFrameSizeCalculation=off
  Vout : Outport  VectorParamsAs1DForOutWhenUnconnected=off
  xdot : Outport  Port=2  VectorParamsAs1DForOutWhenUnconnected=off
  x_new : Outport  Port=3  VectorParamsAs1DForOutWhenUnconnected=off
  Outputs : Outport  Port=4  VectorParamsAs1DForOutWhenUnconnected=off
  Iin : Outport  Port=5  VectorParamsAs1DForOutWhenUnconnected=off
  Heat (W) : Outport  Port=6  VectorParamsAs1DForOutWhenUnconnected=off
  Eff : Outport  Port=7  VectorParamsAs1DForOutWhenUnconnected=off
  wires:
  Temp (Rankine)/1 -> Rankine to Celsius/1, Display/1  "TempIn"
  Rankine to Celsius/1 -> DC - DC Converter/7("T_Ambient "), "Power Loss "/5("T_Ambient ")
  DC - DC Converter/5(switchDyn) -> Bus Creator/1  "switchDyn"
  dt/1 -> DC - DC Converter/4(dt)
  DC - DC Converter/3(x_new) -> Catastrophic Fault Block2/2, Bus Creator/10  "x"
  "Power Loss "/1(" P loss") -> Catastrophic Fault Block5/2, Bus Creator/3, DC - DC Converter/6(P loss)  "P loss"
  d/1 -> DC - DC Converter/3(d), "Power Loss "/3(d)
  x/1 -> DC - DC Converter/2(x)
  DC - DC Converter/4(I_Demanded) -> Product3/2, Catastrophic Fault Block3/2, Bus Creator/2  "Iin"
  DC - DC Converter/2(x_dot) -> Catastrophic Fault Block1/2, Bus Creator/11  "x_dot"
  Iout/1 -> "Power Loss "/2(Iout), DC - DC Converter/5(I_Demand), Switch/2, Bus Creator/5, Product1/1  "Iout"
  DC - DC Converter/1(VOut) -> Catastrophic Fault Block/2, "Power Loss "/4(Vout), Product1/2
  Product1/1 -> Divide1/1, Bus Creator/7, Divide/2  "Pout"
  Product3/1 -> Divide1/2, Bus Creator/6, Divide/1  "Pin"
  "Power Loss "/3(RippleV) -> Bus Creator/9  "Ripple V"
  "Power Loss "/2(RippleI) -> Bus Creator/8  "Ripple I"
  Catastrophic Fault Block/1 -> Vout/1
  [FT] -> Catastrophic Fault Block/1
  [FT] -> Catastrophic Fault Block1/1
  Catastrophic Fault Block1/1 -> xdot/1
  Voltage Catastrophic Fault Block/2 -> DC - DC Converter/1(VIn), "Power Loss "/1(Vin), Product3/1, Bus Creator/4  "Vin"
  Vin/1 -> Voltage Catastrophic Fault Block/2  "Vin"
  FaultToggle/1 -> Voltage Catastrophic Fault Block/1
  Voltage Catastrophic Fault Block/1 -> [FT]
  [FT] -> Catastrophic Fault Block2/1
  Catastrophic Fault Block2/1 -> x_new/1
  [FT] -> Catastrophic Fault Block3/1
  Catastrophic Fault Block3/1 -> Iin/1
  [FT] -> Catastrophic Fault Block4/1
  Bus Creator/1 -> Catastrophic Fault Block4/2
  Catastrophic Fault Block4/1 -> Outputs/1
  [FT] -> Catastrophic Fault Block5/1
  Catastrophic Fault Block5/1 -> Heat (W)/1
  Catastrophic Fault Block6/1 -> Eff/1
  [FT] -> Catastrophic Fault Block6/1
  Switch/1 -> Catastrophic Fault Block6/2
  Divide1/1 -> Switch/1
  Divide/1 -> Switch/3

== system Lib_EMTAT/Components/Physics-Based/Buck Converter ==
  Vin : Inport
  x : Inport  Port=2
  d : Inport  Port=3
  dt : Inport  Port=4
  I_Demand : Inport  Port=5
  T_Ambient : Inport  Port=6  Unit=degC
  FaultToggle : Inport  Port=7  Unit=degC
  Bus Creator : BusCreator  Inputs=11
  Catastrophic Fault Block{,1..6} (7 alike) : $bdroot/Components/Physics-Based/Catastrophic Fault Block  SystemSampleTime=-1  VariantActivationTime=update diagram  Latency=0  AutoFrameSizeCalculation=off
  DC - DC Converter : Subsystem
  Divide : Product  Inputs=*/
  Divide1 : Product  Inputs=*/
  "Power Loss " : Subsystem
  Product1 : Product
  Product3 : Product
  Rankine to Celsius : $bdroot/Components/Physics-Based/Rankine to Celsius  SystemSampleTime=-1  VariantActivationTime=update diagram  Latency=0  AutoFrameSizeCalculation=off
  Switch : Switch  Criteria=u2 > Threshold
  Voltage Catastrophic Fault Block : $bdroot/Components/Physics-Based/Voltage Catastrophic Fault Block  SystemSampleTime=-1  VariantActivationTime=update diagram  Latency=0  AutoFrameSizeCalculation=off
  Vout : Outport  VectorParamsAs1DForOutWhenUnconnected=off
  xdot : Outport  Port=2  VectorParamsAs1DForOutWhenUnconnected=off
  x_new : Outport  Port=3  VectorParamsAs1DForOutWhenUnconnected=off
  Outputs : Outport  Port=4  VectorParamsAs1DForOutWhenUnconnected=off
  I_Demanded : Outport  Port=5  VectorParamsAs1DForOutWhenUnconnected=off
  Heat : Outport  Port=6  VectorParamsAs1DForOutWhenUnconnected=off
  Eff : Outport  Port=7  VectorParamsAs1DForOutWhenUnconnected=off
  wires:
  Voltage Catastrophic Fault Block/2 -> Product3/1, Bus Creator/4, DC - DC Converter/1(VIn), "Power Loss "/1(Vin)  "Vin"
  "Power Loss "/2(RippleI) -> Bus Creator/8  "Ripple I"
  "Power Loss "/3(RippleV) -> Bus Creator/9  "Ripple V"
  DC - DC Converter/1(Vout) -> Catastrophic Fault Block/2, "Power Loss "/4(Vout), Product1/2
  DC - DC Converter/2(x_dot) -> Catastrophic Fault Block1/2, Bus Creator/11  "x_dot"
  DC - DC Converter/4(I_Demanded) -> Catastrophic Fault Block3/2, Bus Creator/2, Product3/2  "Iin"
  x/1 -> DC - DC Converter/2(x)
  d/1 -> "Power Loss "/3(d), DC - DC Converter/3(d)
  "Power Loss "/1(" P loss") -> DC - DC Converter/6(P loss), Catastrophic Fault Block6/2, Bus Creator/3  "P loss"
  DC - DC Converter/3(x_new) -> Catastrophic Fault Block2/2, Bus Creator/10  "x"
  dt/1 -> DC - DC Converter/4(dt)
  DC - DC Converter/5(switchDyn) -> Bus Creator/1  "switchDyn"
  T_Ambient/1 -> Rankine to Celsius/1
  Rankine to Celsius/1 -> "Power Loss "/5("T_Ambient "), DC - DC Converter/7("T_Ambient ")
  [FT] -> Catastrophic Fault Block/1
  Catastrophic Fault Block/1 -> Vout/1
  [FT] -> Catastrophic Fault Block1/1
  Catastrophic Fault Block1/1 -> xdot/1
  [FT] -> Catastrophic Fault Block2/1
  Catastrophic Fault Block2/1 -> x_new/1
  [FT] -> Catastrophic Fault Block3/1
  Catastrophic Fault Block3/1 -> I_Demanded/1
  [FT] -> Catastrophic Fault Block4/1
  Bus Creator/1 -> Catastrophic Fault Block4/2
  Catastrophic Fault Block4/1 -> Outputs/1
  [FT] -> Catastrophic Fault Block6/1
  Catastrophic Fault Block6/1 -> Heat/1
  FaultToggle/1 -> Voltage Catastrophic Fault Block/1
  Catastrophic Fault Block5/1 -> Eff/1
  [FT] -> Catastrophic Fault Block5/1
  Product3/1 -> Divide1/2, Divide/1, Bus Creator/6  "Pin"
  Product1/1 -> Divide1/1, Divide/2, Bus Creator/7  "Pout"
  Divide1/1 -> Switch/1
  Divide/1 -> Switch/3
  I_Demand/1 -> "Power Loss "/2(Iout), Product1/1, Switch/2, Bus Creator/5, DC - DC Converter/5(I_Demand)  "Iout"
  Switch/1 -> Catastrophic Fault Block5/2
  Vin/1 -> Voltage Catastrophic Fault Block/2  "Vin"
  Voltage Catastrophic Fault Block/1 -> [FT]

== system Lib_EMTAT/Components/Physics-Based/Cable Model ==
  note: UPDATE RESISTANCE BASED ON AMBIENT TEMPERATURE CHANGE
  note: GENERAL ELECTRICAL CALCULATIONS
  note: ------------------------------------------------
      | Created by Nathan Butler
      | NASA Glenn Research Center
      | MATLAB R2020b
      | Spring 2021
      | ------------------------------------------------
  Idemand : Inport
  Vin : Inport  Port=2
  Temp : Inport  Port=3
  FaultToggle : Inport  Port=4
  Degredation Factor : Inport  Port=5
  Add : Sum
  Catastrophic Fault Block : $bdroot/Components/Physics-Based/Catastrophic Fault Block  SystemSampleTime=-1  VariantActivationTime=update diagram  Latency=0  AutoFrameSizeCalculation=off
  Catastrophic Fault Block1 : $bdroot/Components/Physics-Based/Catastrophic Fault Block  SystemSampleTime=-1  VariantActivationTime=update diagram  Latency=0  AutoFrameSizeCalculation=off
  Catastrophic Fault Block2 : $bdroot/Components/Physics-Based/Catastrophic Fault Block  SystemSampleTime=-1  VariantActivationTime=update diagram  Latency=0  AutoFrameSizeCalculation=off
  Constant : Constant  Value=alpha
  Constant1 : Constant
  Constant2 : Constant
  Constant3 : Constant  Value=R_init
  Divide : Product  Inputs=**
  I_dmd*Vdrop : Product
  Product : Product
  Product1 : Product
  Product3 : Product
  Rankine to Celsius : $bdroot/Components/Physics-Based/Rankine to Celsius  SystemSampleTime=-1  VariantActivationTime=update diagram  Latency=0  AutoFrameSizeCalculation=off
  Ref Temp (C) : Constant  Value=20
  Subtract1 : Sum  Inputs=+-
  Switch : Switch  Criteria=u2 ~= 0  Threshold=~0
  Vin-Vdrop : Sum  Inputs=+-
  Voltage Catastrophic Fault Block : $bdroot/Components/Physics-Based/Voltage Catastrophic Fault Block  SystemSampleTime=-1  VariantActivationTime=update diagram  Latency=0  AutoFrameSizeCalculation=off
  Idemanded : Outport  VectorParamsAs1DForOutWhenUnconnected=off
  Vout : Outport  Port=2  VectorParamsAs1DForOutWhenUnconnected=off
  Heat : Outport  Port=3  VectorParamsAs1DForOutWhenUnconnected=off
  wires:
  Subtract1/1 -> Product/2  "delta_T"
  Constant/1 -> Product/1
  Product/1 -> Add/2
  Constant1/1 -> Add/1
  Add/1 -> Product1/1  "1+alpha(deltaT)"
  Product1/1 -> Divide/2  "R2"
  Constant3/1 -> Product1/2
  Ref Temp (C)/1 -> Subtract1/2
  Vin-Vdrop/1 -> Catastrophic Fault Block1/2
  Idemand/1 -> Product3/1, Catastrophic Fault Block/2, I_dmd*Vdrop/2
  [R] -> Product3/2
  Product3/1 -> I_dmd*Vdrop/1, Vin-Vdrop/2  "VDrop"
  Temp/1 -> Rankine to Celsius/1
  Rankine to Celsius/1 -> Subtract1/1
  Catastrophic Fault Block/1 -> Idemanded/1
  [FT] -> Catastrophic Fault Block/1
  [FT] -> Catastrophic Fault Block1/1
  [FT] -> Catastrophic Fault Block2/1
  I_dmd*Vdrop/1 -> Catastrophic Fault Block2/2
  Catastrophic Fault Block2/1 -> Heat/1
  Catastrophic Fault Block1/1 -> Vout/1
  Vin/1 -> Voltage Catastrophic Fault Block/2
  Voltage Catastrophic Fault Block/2 -> Vin-Vdrop/1
  Voltage Catastrophic Fault Block/1 -> [FT]
  FaultToggle/1 -> Voltage Catastrophic Fault Block/1
  Constant2/1 -> Switch/3
  Switch/1 -> Divide/1
  Degredation Factor/1 -> Switch/2, Switch/1
  Divide/1 -> [R]

== system Lib_EMTAT/Components/Physics-Based/Catastrophic Fault Block ==
  Fault Toggle : Inport
  Inport Value : Inport  Port=2
  Display{,1..3} (4 alike) : Display
  OR1 : Logic  Operator=OR  IconShape=distinctive  AllPortsSameDT=off  OutDataTypeStr=boolean
  Relational Operator : RelationalOperator  Operator=isInf  OutDataTypeStr=boolean  RndMeth=Simplest
  Relational Operator3 : RelationalOperator  Operator=isNaN  OutDataTypeStr=boolean  RndMeth=Simplest
  Switch1 : Switch  Criteria=u2 > Threshold
  Switch2 : Switch  Criteria=u2 > Threshold
  Zero1 : Constant  Value=0
  Zero2 : Constant  Value=0
  Outport Value : Outport
  wires:
  Fault Toggle/1 -> Switch2/2
  Zero2/1 -> Switch1/1
  Zero1/1 -> Switch2/1
  Inport Value/1 -> Switch2/3
  OR1/1 -> Display2/1, Switch1/2
  Relational Operator3/1 -> OR1/2
  Relational Operator/1 -> OR1/1
  Switch1/1 -> Display1/1, Outport Value/1
  Switch2/1 -> Display3/1, Display/1, Switch1/3, Relational Operator3/1, Relational Operator/1

== system Lib_EMTAT/Components/Physics-Based/Degradation Input Block ==
  Degradation Input Value : Constant  Value=component_degradation_input
  Disp Degradation Input : Display
  Disp Original Degradation Factor : Display
  Exp : Math  Operator=10^u  SaturateOnIntegerOverflow=on
  Reciprocal : Product  Inputs=/
  Degradation Factor : Outport
  Degradation Input : Outport  Port=2
  wires:
  Degradation Input Value/1 -> Exp/1, Degradation Input/1, Disp Degradation Input/1
  Exp/1 -> Reciprocal/1
  Reciprocal/1 -> Disp Original Degradation Factor/1, Degradation Factor/1

== system Lib_EMTAT/Components/Physics-Based/Degradation Parameter Multiplier ==
  Parameter Adjustment : Inport
  Display{,1..4} (5 alike) : Display
  Exp1 : Math  Operator=10^u  SaturateOnIntegerOverflow=on
  Product3 : Product
  Product4 : Product
  Adjusted Degradation Factor : Outport
  wires:
  Parameter Adjustment/1 -> Product4/2
  Product4/1 -> Display3/1, Exp1/1
  [component_DI] -> Display4/1, Product4/1
  Product3/1 -> Display/1, Adjusted Degradation Factor/1
  Exp1/1 -> Display2/1, Product3/1
  [component_DF] -> Display1/1, Product3/2
